simulink model "RTDinamicInvPID"  (R2018a)
settings: Solver=VariableStepAuto  StartTime=0.0  StopTime=3  RelTol=1e-3
settings Model: Creator=ilier  LastModifiedBy=ilier

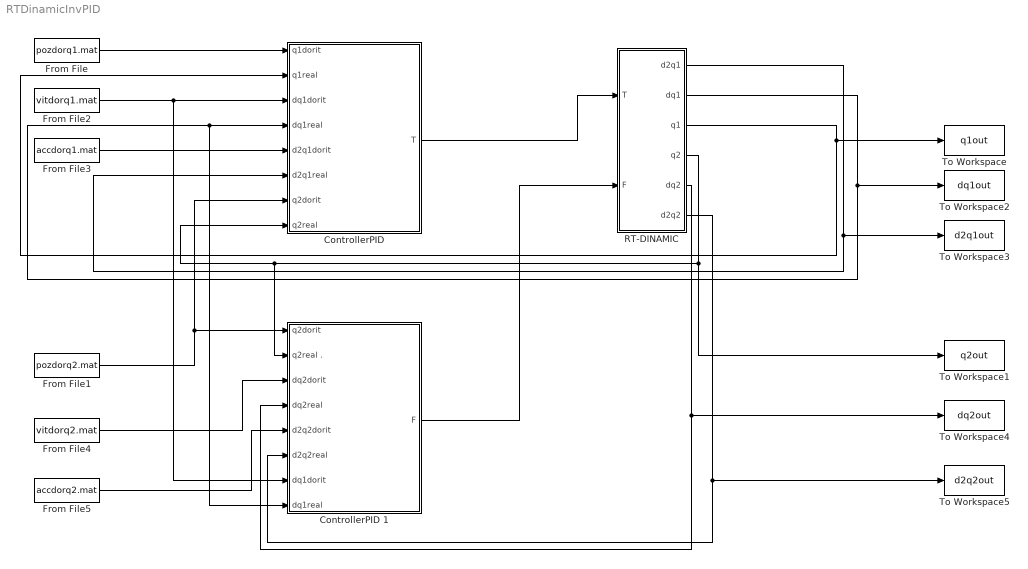
== system RTDinamicInvPID ==
  "ControllerPID " : Subsystem
  ControllerPID 1 : Subsystem
  From File : FromFile  FileName=pozdorq1.mat  SampleTime=0
  From File1 : FromFile  FileName=pozdorq2.mat  SampleTime=0
  From File2 : FromFile  FileName=vitdorq1.mat  SampleTime=0
  From File3 : FromFile  FileName=accdorq1.mat  SampleTime=0
  From File4 : FromFile  FileName=vitdorq2.mat  SampleTime=0
  From File5 : FromFile  FileName=accdorq2.mat  SampleTime=0
  RT-DINAMIC : Subsystem
  To Workspace : ToWorkspace  VariableName=q1out  SaveFormat=Timeseries  SampleTime=-1
  To Workspace1 : ToWorkspace  VariableName=q2out  SaveFormat=Timeseries  SampleTime=-1
  To Workspace2 : ToWorkspace  VariableName=dq1out  SaveFormat=Timeseries  SampleTime=-1
  To Workspace3 : ToWorkspace  VariableName=d2q1out  SaveFormat=Timeseries  SampleTime=-1
  To Workspace4 : ToWorkspace  VariableName=dq2out  SaveFormat=Timeseries  SampleTime=-1
  To Workspace5 : ToWorkspace  VariableName=d2q2out  SaveFormat=Timeseries  SampleTime=-1
  wires:
  RT-DINAMIC/5(dq2) -> To Workspace4/1, ControllerPID 1/4(dq2real)
  From File5/1 -> ControllerPID 1/5(d2q2dorit)
  RT-DINAMIC/1(d2q1) -> "ControllerPID "/6("d2q1real "), To Workspace3/1
  RT-DINAMIC/6(d2q2) -> To Workspace5/1, ControllerPID 1/6("d2q2real ")
  From File2/1 -> ControllerPID 1/7("dq1dorit "), "ControllerPID "/3("dq1dorit ")
  From File4/1 -> ControllerPID 1/3("dq2dorit ")
  ControllerPID 1/1(F) -> RT-DINAMIC/2(F)
  "ControllerPID "/1(T) -> RT-DINAMIC/1(T)
  From File1/1 -> ControllerPID 1/1(q2dorit), "ControllerPID "/7("q2dorit ")
  RT-DINAMIC/3(q1) -> To Workspace/1, "ControllerPID "/2(q1real)
  RT-DINAMIC/2(dq1) -> To Workspace2/1, ControllerPID 1/8(dq1real), "ControllerPID "/4(dq1real)
  From File/1 -> "ControllerPID "/1(q1dorit)
  From File3/1 -> "ControllerPID "/5(d2q1dorit)
  RT-DINAMIC/4(q2) -> To Workspace1/1, ControllerPID 1/2(q2real .), "ControllerPID "/8(q2real)

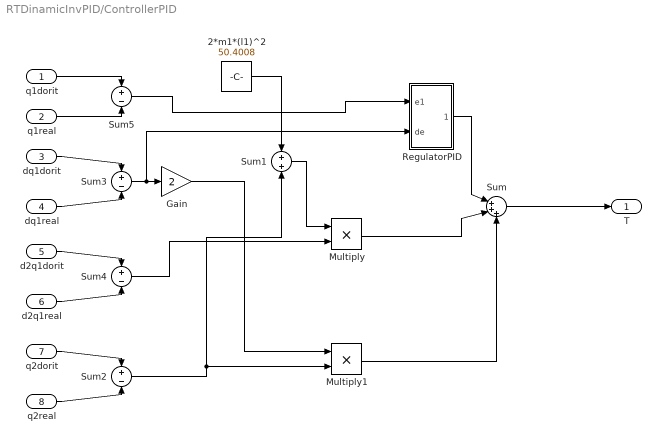
== system RTDinamicInvPID/ControllerPID  ==
  q1dorit : Inport
  q1real : Inport  Port=2
  "dq1dorit " : Inport  Port=3
  dq1real : Inport  Port=4
  d2q1dorit : Inport  Port=5
  "d2q1real " : Inport  Port=6
  "q2dorit " : Inport  Port=7
  q2real : Inport  Port=8
  2*m1*(l1)^2 : Constant  Value=50.4008
  Gain : Gain  Gain=2
  Multiply : Product
  Multiply1 : Product
  RegulatorPID : Subsystem
  Sum : Sum  Inputs=|+++
  Sum1 : Sum
  Sum{2..5} (4 alike) : Sum  Inputs=+-
  T : Outport
  wires:
  Sum1/1 -> Multiply/1
  2*m1*(l1)^2/1 -> Sum1/1
  q1dorit/1 -> Sum5/1
  "q2dorit "/1 -> Sum2/1
  dq1real/1 -> Sum3/2
  Sum2/1 -> Multiply1/2, Sum1/2
  RegulatorPID/1(u*1) -> Sum/1
  Sum/1 -> T/1
  Gain/1 -> Multiply1/1
  Sum3/1 -> RegulatorPID/2(de), Gain/1
  Sum5/1 -> RegulatorPID/1(e1)
  q2real/1 -> Sum2/2
  "d2q1real "/1 -> Sum4/2
  "dq1dorit "/1 -> Sum3/1
  Sum4/1 -> Multiply/2
  q1real/1 -> Sum5/2
  d2q1dorit/1 -> Sum4/1
  Multiply/1 -> Sum/2
  Multiply1/1 -> Sum/3

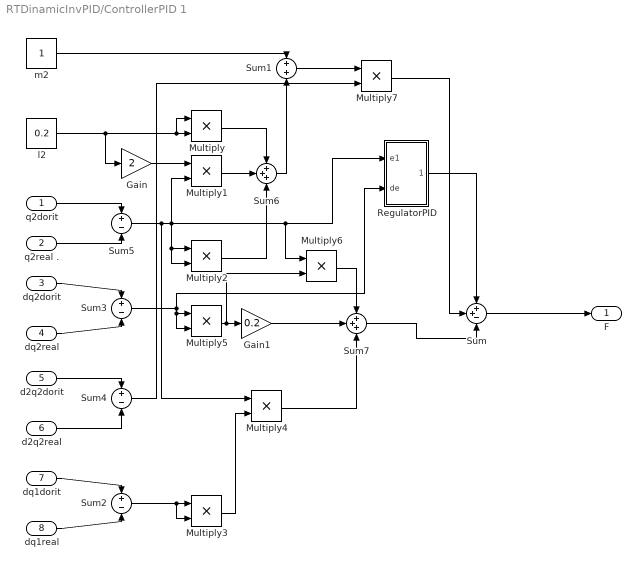
== system RTDinamicInvPID/ControllerPID 1 ==
  q2dorit : Inport
  q2real . : Inport  Port=2
  "dq2dorit " : Inport  Port=3
  dq2real : Inport  Port=4
  d2q2dorit : Inport  Port=5
  "d2q2real " : Inport  Port=6
  "dq1dorit " : Inport  Port=7
  dq1real : Inport  Port=8
  Gain : Gain  Gain=2
  Gain1 : Gain  Gain=0.2
  Multiply{,1..7} (8 alike) : Product
  RegulatorPID : Subsystem
  Sum : Sum  Inputs=++-
  Sum1 : Sum
  Sum{2..5} (4 alike) : Sum  Inputs=+-
  Sum6 : Sum  Inputs=+++
  Sum7 : Sum  Inputs=+++
  l2 : Constant  Value=0.2
  m2 : Constant
  F : Outport
  wires:
  q2dorit/1 -> Sum5/1
  "dq1dorit "/1 -> Sum2/1
  dq2real/1 -> Sum3/2
  Sum2/1 -> Multiply3/2, Multiply3/1
  RegulatorPID/1(u*1) -> Sum/1
  Sum/1 -> F/1
  dq1real/1 -> Sum2/2
  "d2q2real "/1 -> Sum4/2
  "dq2dorit "/1 -> Sum3/1
  q2real ./1 -> Sum5/2
  d2q2dorit/1 -> Sum4/1
  m2/1 -> Sum1/1
  Multiply/1 -> Sum6/1
  l2/1 -> Multiply/1, Multiply/2, Gain/1
  Gain/1 -> Multiply1/1
  Sum5/1 -> RegulatorPID/1(e1), Multiply6/1, Multiply2/1, Multiply2/2, Multiply1/2, Multiply4/1
  Multiply1/1 -> Sum6/2
  Multiply2/1 -> Sum6/3
  Sum6/1 -> Sum1/2
  Multiply3/1 -> Multiply4/2
  Multiply4/1 -> Sum7/3
  Sum3/1 -> RegulatorPID/2(de), Multiply5/2, Multiply5/1
  Multiply5/1 -> Multiply6/2, Gain1/1
  Gain1/1 -> Sum7/2
  Multiply6/1 -> Sum7/1
  Sum7/1 -> Sum/3
  Sum1/1 -> Multiply7/1
  Sum4/1 -> Multiply7/2
  Multiply7/1 -> Sum/2

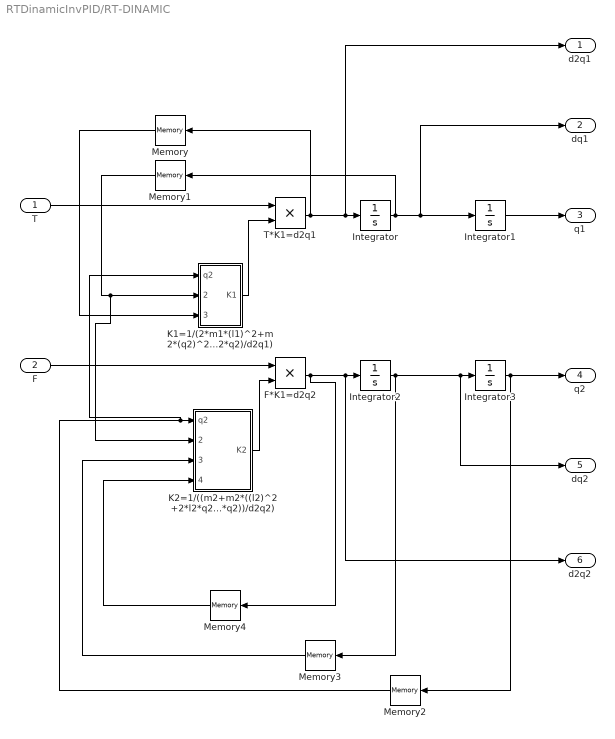
== system RTDinamicInvPID/RT-DINAMIC ==
  T : Inport
  F : Inport  Port=2
  F*K1=d2q2 : Product
  Integrator{,1..3} (4 alike) : Integrator
  K1=1/(2*m1*(l1)^2+m2*(q2)^2+(2*dq1*m2*q2)/d2q1) : Subsystem
  K2=1/((m2+m2*((l2)^2+2*l2*q2+(q2)^2)) -(m2*((dq1)^2*q2+(dq2)^2*l2+(dq2)^2*q2))/d2q2) : Subsystem
  Memory{,1..4} (5 alike) : Memory
  T*K1=d2q1 : Product
  d2q1 : Outport
  dq1 : Outport  Port=2
  q1 : Outport  Port=3
  q2 : Outport  Port=4
  dq2 : Outport  Port=5
  d2q2 : Outport  Port=6
  wires:
  F/1 -> F*K1=d2q2/1
  K1=1/(2*m1*(l1)^2+m2*(q2)^2+(2*dq1*m2*q2)/d2q1)/1(K1) -> T*K1=d2q1/2
  T/1 -> T*K1=d2q1/1
  T*K1=d2q1/1 -> Memory/1, d2q1/1, Integrator/1
  Integrator/1 -> Memory1/1, dq1/1, Integrator1/1
  Integrator1/1 -> q1/1
  Memory/1 -> K1=1/(2*m1*(l1)^2+m2*(q2)^2+(2*dq1*m2*q2)/d2q1)/3(d2q1)
  Memory1/1 -> K2=1/((m2+m2*((l2)^2+2*l2*q2+(q2)^2)) -(m2*((dq1)^2*q2+(dq2)^2*l2+(dq2)^2*q2))/d2q2)/2(derivQ1), K1=1/(2*m1*(l1)^2+m2*(q2)^2+(2*dq1*m2*q2)/d2q1)/2(dq1)
  K2=1/((m2+m2*((l2)^2+2*l2*q2+(q2)^2)) -(m2*((dq1)^2*q2+(dq2)^2*l2+(dq2)^2*q2))/d2q2)/1(K2) -> F*K1=d2q2/2
  F*K1=d2q2/1 -> Memory4/1, d2q2/1, Integrator2/1
  Integrator2/1 -> Memory3/1, dq2/1, Integrator3/1
  Integrator3/1 -> Memory2/1, q2/1
  Memory2/1 -> K1=1/(2*m1*(l1)^2+m2*(q2)^2+(2*dq1*m2*q2)/d2q1)/1("q2 "), K2=1/((m2+m2*((l2)^2+2*l2*q2+(q2)^2)) -(m2*((dq1)^2*q2+(dq2)^2*l2+(dq2)^2*q2))/d2q2)/1(q2)
  Memory3/1 -> K2=1/((m2+m2*((l2)^2+2*l2*q2+(q2)^2)) -(m2*((dq1)^2*q2+(dq2)^2*l2+(dq2)^2*q2))/d2q2)/3(derivQ2)
  Memory4/1 -> K2=1/((m2+m2*((l2)^2+2*l2*q2+(q2)^2)) -(m2*((dq1)^2*q2+(dq2)^2*l2+(dq2)^2*q2))/d2q2)/4(deriv2Q2)

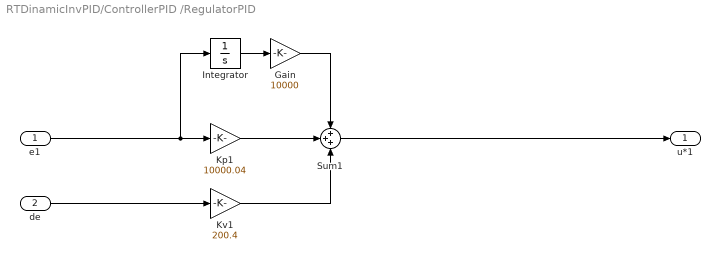
== system RTDinamicInvPID/ControllerPID /RegulatorPID ==
  e1 : Inport
  de : Inport  Port=2
  Gain : Gain  Gain=10000
  Integrator : Integrator
  Kp1 : Gain  Gain=10000.04
  Kv1 : Gain  Gain=200.4
  Sum1 : Sum  Inputs=+++
  u*1 : Outport
  wires:
  de/1 -> Kv1/1
  e1/1 -> Integrator/1, Kp1/1
  Kv1/1 -> Sum1/3
  Kp1/1 -> Sum1/2
  Sum1/1 -> u*1/1
  Gain/1 -> Sum1/1
  Integrator/1 -> Gain/1

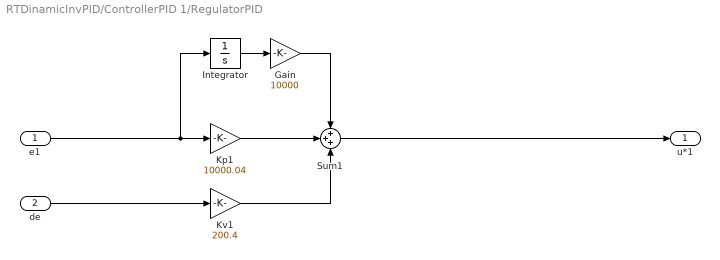
== system RTDinamicInvPID/ControllerPID 1/RegulatorPID ==
  e1 : Inport
  de : Inport  Port=2
  Gain : Gain  Gain=10000
  Integrator : Integrator
  Kp1 : Gain  Gain=10000.04
  Kv1 : Gain  Gain=200.4
  Sum1 : Sum  Inputs=+++
  u*1 : Outport
  wires:
  de/1 -> Kv1/1
  e1/1 -> Integrator/1, Kp1/1
  Kv1/1 -> Sum1/3
  Kp1/1 -> Sum1/2
  Sum1/1 -> u*1/1
  Gain/1 -> Sum1/1
  Integrator/1 -> Gain/1

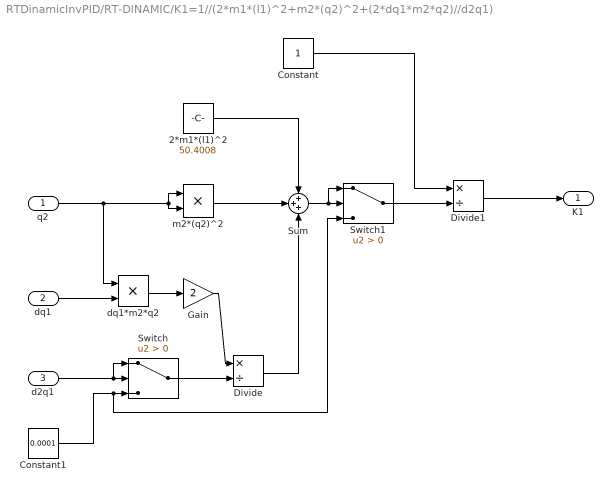
== system RTDinamicInvPID/RT-DINAMIC/K1=1//(2*m1*(l1)^2+m2*(q2)^2+(2*dq1*m2*q2)//d2q1) ==
  "q2 " : Inport
  dq1 : Inport  Port=2
  d2q1 : Inport  Port=3
  2*m1*(l1)^2 : Constant  Value=50.4008
  Constant : Constant
  Constant1 : Constant  Value=0.0001
  Divide : Product  Inputs=*/
  Divide1 : Product  Inputs=*/
  Gain : Gain  Gain=2
  Sum : Sum  Inputs=+++
  Switch : Switch  Criteria=u2 > Threshold
  Switch1 : Switch  Criteria=u2 > Threshold
  dq1*m2*q2 : Product
  m2*(q2)^2 : Product
  K1 : Outport
  wires:
  "q2 "/1 -> dq1*m2*q2/1, m2*(q2)^2/2, m2*(q2)^2/1
  2*m1*(l1)^2/1 -> Sum/1
  Sum/1 -> Switch1/1, Switch1/2
  m2*(q2)^2/1 -> Sum/2
  Divide/1 -> Sum/3
  dq1/1 -> dq1*m2*q2/2
  dq1*m2*q2/1 -> Gain/1
  Constant/1 -> Divide1/1
  Gain/1 -> Divide/1
  Divide1/1 -> K1/1
  Switch/1 -> Divide/2
  d2q1/1 -> Switch/1, Switch/2
  Constant1/1 -> Switch1/3, Switch/3
  Switch1/1 -> Divide1/2

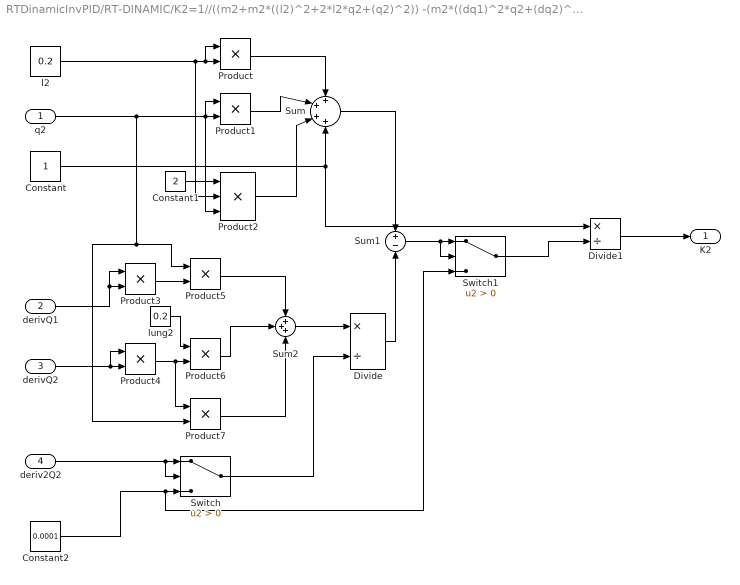
== system RTDinamicInvPID/RT-DINAMIC/K2=1//((m2+m2*((l2)^2+2*l2*q2+(q2)^2)) -(m2*((dq1)^2*q2+(dq2)^2*l2+(dq2)^2*q2))//d2q2) ==
  q2 : Inport
  derivQ1 : Inport  Port=2
  derivQ2 : Inport  Port=3
  deriv2Q2 : Inport  Port=4
  Constant : Constant
  Constant1 : Constant  Value=2
  Constant2 : Constant  Value=0.0001
  Divide : Product  Inputs=*/
  Divide1 : Product  Inputs=*/
  Product{,1,3..7} (7 alike) : Product
  Product2 : Product  Inputs=3
  Sum : Sum  Inputs=++++
  Sum1 : Sum  Inputs=+-
  Sum2 : Sum  Inputs=+++
  Switch : Switch  Criteria=u2 > Threshold
  Switch1 : Switch  Criteria=u2 > Threshold
  l2 : Constant  Value=0.2
  lung2 : Constant  Value=0.2
  K2 : Outport
  wires:
  Product5/1 -> Sum2/1
  q2/1 -> Product5/1, Product7/2, Product1/1, Product1/2, Product2/3
  Product1/1 -> Sum/2
  Sum2/1 -> Divide/1
  derivQ1/1 -> Product3/2, Product3/1
  Product4/1 -> Product7/1, Product6/2
  Product6/1 -> Sum2/2
  deriv2Q2/1 -> Switch/2, Switch/1
  l2/1 -> Product/1, Product/2, Product2/2
  Product7/1 -> Sum2/3
  Sum/1 -> Sum1/1
  Divide/1 -> Sum1/2
  Divide1/1 -> K2/1
  derivQ2/1 -> Product4/1, Product4/2
  Constant/1 -> Divide1/1, Sum/4
  lung2/1 -> Product6/1
  Constant1/1 -> Product2/1
  Product3/1 -> Product5/2
  Switch/1 -> Divide/2
  Product/1 -> Sum/1
  Constant2/1 -> Switch1/3, Switch/3
  Product2/1 -> Sum/3
  Sum1/1 -> Switch1/2, Switch1/1
  Switch1/1 -> Divide1/2
